simulink model "sampleModel273"  (R2021b)
settings: Solver=VariableStepAuto  StartTime=0.0  StopTime=10.0  RelTol=1e-3
undefined symbols (not defined in the file or in its folder): DiscIntNeverNeededParam
libraries: simulink x13
settings Model: Creator=user  LastModifiedBy=user

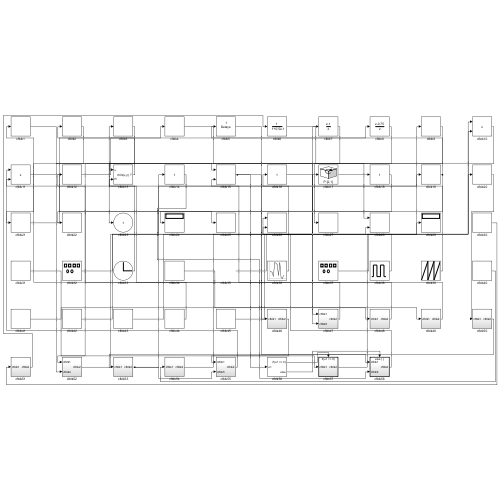
[thumbnail: Simulink's stored preview of the top-level diagram]
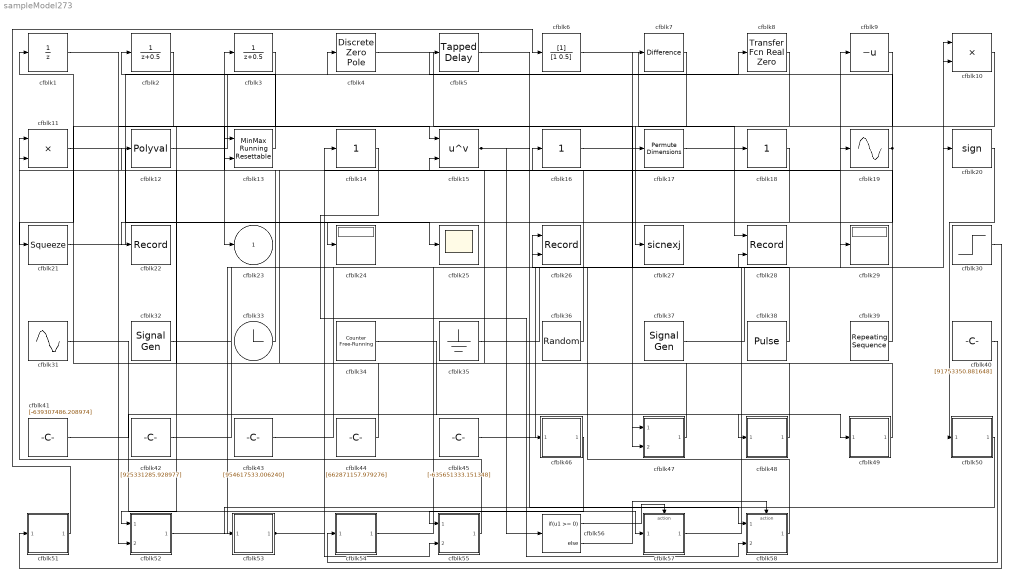
== system sampleModel273 ==
  cfblk1 : UnitDelay  HasFrameUpgradeWarning=on
  cfblk10 : Product
  cfblk11 : Product
  cfblk12 : Polyval  Coefs=[ +2.081618890e-019, -1.441693666e-014, +4.719686976e-010, -8.536869453e-006, +1.621573104e-001, -8.087801117e+001 ]
  cfblk13 : simulink/Math Operations/MinMax Running Resettable  Function=min  vinit=0.0
  cfblk14 : simulink/Math Operations/Slider Gain  gain=1  low=0  high=2
  cfblk15 : Math  Operator=pow  SaturateOnIntegerOverflow=on
  cfblk16 : simulink/Math Operations/Slider Gain  gain=1  low=0  high=2
  cfblk17 : PermuteDimensions
  cfblk18 : simulink/Math Operations/Slider Gain  gain=1  low=0  high=2
  cfblk19 : Sin  TimeSource=Use external signal  SampleTime=0
  cfblk2 : DiscreteTransferFcn  SampleTime=1
  cfblk20 : Signum
  cfblk21 : Squeeze
  cfblk22 : Record  FileSettingsInternal="{\"entries\":[{\"content\":{\"excelSettings\":{\"content\":{},\"type\":\"Streamout.ExcelSettings\"}},\"type\":\"Streamout.FileSettingStorage\",\"uuid\":\"1786dd08-d3d1-48fd-88f3-6c9c5e3b2244\"}],\"packageUris\":[\"http://schema.mathworks.com/mf0/streamout_blocks/R2020a\"],\"version\":\"1.0\"}"  SignalsInternal="{\"entries\":[{\"content\":{\"signals\":[{\"content\":{\"blockPath\":[\"sampleModel273/cfblk22\"],\"channel\":[],\"dimensions\":[1,1],\"domain\":\"sampleModel273/cfblk22\",\"lineColor\":\"#ff13a6\",\"plots\":[1],\"port\":1,\"sid\":[\"\"],\"signalID\":11389,\"signalName\":\"cfblk18\"},\"type\":\"RecordBlkView.Signal\",\"uuid\":\"44d7af05-e021-4219-85f4-b2264b388561\"}]},\"type\":\"RecordBlkView.InputSignals\",\"uuid\":\"1305e598-0f40-4dae-bf49-06488a9adac4\"}],\"packageUris\":[\"http://schema.mathworks.com/mf0/streamout_blocks/R2020a\"],\"version\":\"1.0\"}"  VisualizationBindings="{\"sparklinesplugin\":{\"info\":[{\"bindingParametersList\":[],\"subplotID\":1}]}}"
  cfblk24 : Display
  cfblk25 : Scope
  cfblk26 : Record  FileSettingsInternal="{\"entries\":[{\"content\":{\"excelSettings\":{\"content\":{},\"type\":\"Streamout.ExcelSettings\"}},\"type\":\"Streamout.FileSettingStorage\",\"uuid\":\"c9907c03-a1b4-46c3-905a-7ea5945ed0d3\"}],\"packageUris\":[\"http://schema.mathworks.com/mf0/streamout_blocks/R2020a\"],\"version\":\"1.0\"}"  Layout=[1 1]  SignalsInternal="{\"entries\":[{\"content\":{\"signals\":[{\"content\":{\"blockPath\":[\"sampleModel273/cfblk26\"],\"channel\":[],\"dimensions\":[1],\"domain\":\"sampleModel273/cfblk26\",\"lineColor\":\"#a2142f\",\"plots\":[1],\"port\":1,\"sid\":[\"\"],\"signalID\":11373,\"signalName\":\"cfblk38\"},\"type\":\"RecordBlkView.Signal\",\"uuid\":\"10f35443-25b8-4ed5-9519-77cd749e2a49\"},{\"content\":{\"blockPath\":[\"sampleModel273/cfblk26\"],\"channel\":[],\"dimensions\":[1],\"domain\":\"sampleModel273/cfblk26\",\"lineColor\":\"#139fff\",\"plots\":[1],\"port\":2,\"sid\":[\"\"],\"signalID\":11377,\"signalName\":\"cfblk58\"},\"type\":\"RecordBlkView.Signal\",\"uuid\":\"581304bf-ecf3-443c-9df5-bbc4588b99e1\"}]},\"type\":\"RecordBlkView.InputSignals\",\"uuid\":\"7f34d2d8-bb93-478d-8761-c598979a6e05\"}],\"packageUris\":[\"http://schema.mathworks.com/mf0/streamout_blocks/R2020a\"],\"version\":\"1.0\"}"  VisualizationBindings="{\"xyplotplugin\":{\"info\":[{\"series\":[{\"bindingParametersList\":[{\"parameter\":\"X-Axis\",\"signalID\":11373,\"signalName\":\"cfblk38\"},{\"parameter\":\"Y-Axis\",\"signalID\":11377,\"signalName\":\"cfblk58\"}],\"seriesID\":34757}],\"subplotID\":1}]}}"  CompatibilityTag=XY
  cfblk27 : ToWorkspace  VariableName=sicnexj  SaveFormat=Timeseries  SampleTime=-1
  cfblk28 : Record  FileSettingsInternal="{\"entries\":[{\"content\":{\"excelSettings\":{\"content\":{},\"type\":\"Streamout.ExcelSettings\"}},\"type\":\"Streamout.FileSettingStorage\",\"uuid\":\"f11b4837-361d-47ed-bc23-be4c68ae3fbc\"}],\"packageUris\":[\"http://schema.mathworks.com/mf0/streamout_blocks/R2020a\"],\"version\":\"1.0\"}"  Layout=[1 1]  SignalsInternal="{\"entries\":[{\"content\":{\"signals\":[{\"content\":{\"blockPath\":[\"sampleModel273/cfblk28\"],\"channel\":[],\"dimensions\":[1],\"domain\":\"sampleModel273/cfblk28\",\"lineColor\":\"#a2142f\",\"plots\":[1],\"port\":1,\"sid\":[\"\"],\"signalID\":11381,\"signalName\":\"cfblk6\"},\"type\":\"RecordBlkView.Signal\",\"uuid\":\"39c39639-ba01-4672-b896-9cb9c6ecd09e\"},{\"content\":{\"blockPath\":[\"sampleModel273/cfblk28\"],\"channel\":[],\"dimensions\":[1],\"domain\":\"sampleModel273/cfblk28\",\"lineColor\":\"#139fff\",\"plots\":[1],\"port\":2,\"sid\":[\"\"],\"signalID\":11385,\"signalName\":\"cfblk43\"},\"type\":\"RecordBlkView.Signal\",\"uuid\":\"3ede6f01-830a-4ce5-9876-616c533c0d69\"}]},\"type\":\"RecordBlkView.InputSignals\",\"uuid\":\"89d49a1c-fe7b-4ffb-9ac6-606c9b0ce345\"}],\"packageUris\":[\"http://schema.mathworks.com/mf0/streamout_blocks/R2020a\"],\"version\":\"1.0\"}"  VisualizationBindings="{\"xyplotplugin\":{\"info\":[{\"series\":[{\"bindingParametersList\":[{\"parameter\":\"X-Axis\",\"signalID\":11381,\"signalName\":\"cfblk6\"},{\"parameter\":\"Y-Axis\",\"signalID\":11385,\"signalName\":\"cfblk43\"}],\"seriesID\":55614}],\"subplotID\":1}]}}"  CompatibilityTag=XY
  cfblk29 : Display
  cfblk3 : DiscreteTransferFcn  SampleTime=1
  cfblk30 : Step  Time=[48.000000]  Before=[117438544.028774]  After=[817897715.184338]  SampleTime=0
  cfblk31 : Sin  Amplitude=[629555870.349999]  Bias=[755274726.941135]  SampleTime=0
  cfblk32 : SignalGenerator  WaveForm=square  Amplitude=[-783473337.137861]
  cfblk33 : Clock
  cfblk34 : simulink/Sources/Counter Free-Running  NumBits=[52.000000]  tsamp=-1
  cfblk35 : Ground
  cfblk36 : RandomNumber  Mean=[98921.584735]  Variance=[34184.174299]  Seed=[249651186.000000]  SampleTime=0.1
  cfblk37 : SignalGenerator  Amplitude=[196507773.243477]
  cfblk38 : DiscretePulseGenerator  PulseType=Time based  Amplitude=[376878024.596685]  Period=[65768725.640575]  PulseWidth=5  PhaseDelay=[3.000000]
  cfblk39 : simulink/Sources/Repeating Sequence  rep_seq_t=[0 2]  rep_seq_y=[-584950579.786823, 340676402.746707]
  cfblk4 : DiscreteZeroPole  Poles=[0 0.5]  Gain=1
  cfblk40 : Constant  Value=[91753350.881648]  SampleTime=1
  cfblk41 : Constant  Value=[-639307486.208974]  SampleTime=1
  cfblk42 : Constant  Value=[925331285.928977]  SampleTime=1
  cfblk43 : Constant  Value=[954617533.006240]  SampleTime=1
  cfblk44 : Constant  Value=[662871157.979276]  SampleTime=1
  cfblk45 : Constant  Value=[-635651333.151348]  SampleTime=1
  cfblk46 : Subsystem
  cfblk47 : Subsystem
  cfblk48 : Subsystem
  cfblk49 : Subsystem
  cfblk5 : simulink/Discrete/Tapped Delay  vinit=0.0  samptime=-1  NumDelays=1  DelayOrder=Oldest  includeCurrent=off
  cfblk50 : Subsystem
  cfblk51 : Subsystem
  cfblk52 : Subsystem
  cfblk53 : Subsystem
  cfblk54 : Subsystem
  cfblk55 : Subsystem
  cfblk56 : If  IfExpression=u1 >= 0  SampleTime=1
  cfblk57 : Subsystem  TreatAsAtomicUnit=on
  cfblk58 : Subsystem  TreatAsAtomicUnit=on
  cfblk6 : DiscreteFilter  SampleTime=1
  cfblk7 : simulink/Discrete/Difference  ICPrevInput=0.0  OutMin=[]  OutMax=[]  OutDataTypeStr=Inherit: Inherit via back propagation  OutDataType=fixdt(1, 16)  OutScaling=2^-10  DoSatur=off
  cfblk8 : simulink/Discrete/Transfer Fcn Real Zero  ZeroZ=0.75  ICPrevInput=0.0  DoSatur=off
      settings: SourceProductBaseCode=SL
  cfblk9 : UnaryMinus
  cfblk23 : Outport
  wires:
  cfblk8/1 -> cfblk23/1
  cfblk36/1 -> cfblk16/1
  cfblk19/1 -> cfblk24/1, cfblk5/1
  cfblk55/1(cfblk2) -> cfblk11/1
  cfblk57/1(cfblk2) -> cfblk10/1
  cfblk9/1 -> cfblk21/1
  cfblk17/1 -> cfblk18/1
  cfblk44/1 -> cfblk1/1
  cfblk21/1 -> cfblk4/1
  cfblk15/1 -> cfblk58/1(cfblk1), cfblk56/1
  cfblk12/1 -> cfblk8/1
  cfblk14/1 -> cfblk58/2(cfblk5)
  cfblk33/1 -> cfblk3/1
  cfblk37/1 -> cfblk9/1
  cfblk11/1 -> cfblk25/1
  cfblk10/1 -> cfblk27/1
  cfblk20/1 -> cfblk50/1(cfblk1)
  cfblk13/1 -> cfblk2/1
  cfblk52/1(cfblk2) -> cfblk14/1
  cfblk18/1 -> cfblk22/1
  cfblk3/1 -> cfblk52/1(cfblk1)
  cfblk1/1 -> cfblk15/1
  cfblk54/1(cfblk2) -> cfblk10/2
  cfblk35/1 -> cfblk17/1
  cfblk38/1 -> cfblk26/1
  cfblk2/1 -> cfblk52/2(cfblk4)
  cfblk7/1 -> cfblk13/1
  cfblk40/1 -> cfblk54/1(cfblk1)
  cfblk50/1(cfblk2) -> cfblk53/1(cfblk1)
  cfblk6/1 -> cfblk28/1
  cfblk48/1(cfblk2) -> cfblk15/2
  cfblk53/1(cfblk2) -> cfblk19/1, cfblk55/2(cfblk5)
  cfblk45/1 -> cfblk29/1
  cfblk5/1 -> cfblk46/1(cfblk1)
  cfblk42/1 -> cfblk7/1
  cfblk31/1 -> cfblk57/1(cfblk1)
  cfblk41/1 -> cfblk48/1(cfblk1)
  cfblk34/1 -> cfblk49/1(cfblk1)
  cfblk47/1(cfblk2) -> cfblk12/1
  cfblk43/1 -> cfblk28/2
  cfblk58/1(cfblk2) -> cfblk26/2
  cfblk30/1 -> cfblk51/1(cfblk1)
  cfblk32/1 -> cfblk20/1
  cfblk39/1 -> cfblk11/2
  cfblk49/1(cfblk2) -> cfblk13/2
  cfblk16/1 -> cfblk47/1(cfblk1)
  cfblk46/1(cfblk2) -> cfblk55/1(cfblk1)
  cfblk4/1 -> cfblk47/2(cfblk5)
  cfblk51/1(cfblk2) -> cfblk6/1
  cfblk56/1 -> cfblk57/Action
  cfblk56/2 -> cfblk58/Action

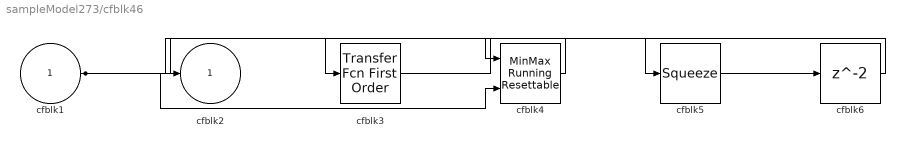
== system sampleModel273/cfblk46 ==
  cfblk1 : Inport
  cfblk3 : simulink/Discrete/Transfer Fcn First Order  PoleZ=0.95  ICPrevOutput=0.0  DoSatur=off
  cfblk4 : simulink/Math Operations/MinMax Running Resettable  Function=min  vinit=0.0
  cfblk5 : Squeeze
  cfblk6 : Delay  SampleTime=1
  cfblk2 : Outport
  wires:
  cfblk3/1 -> cfblk5/1
  cfblk1/1 -> cfblk4/1, cfblk4/2
  cfblk4/1 -> cfblk2/1
  cfblk5/1 -> cfblk6/1
  cfblk6/1 -> cfblk3/1

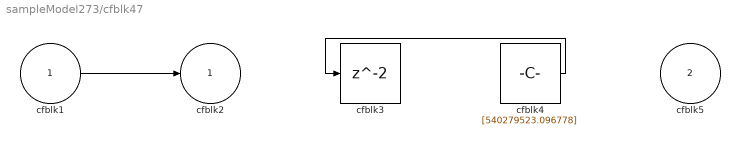
== system sampleModel273/cfblk47 ==
  cfblk1 : Inport
  cfblk5 : Inport  Port=2
  cfblk3 : Delay  SampleTime=1
  cfblk4 : Constant  Value=[540279523.096778]  SampleTime=1
  cfblk2 : Outport
  wires:
  cfblk4/1 -> cfblk3/1
  cfblk1/1 -> cfblk2/1

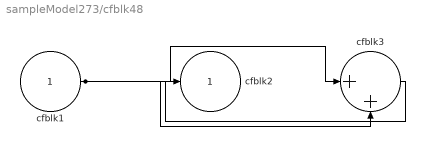
== system sampleModel273/cfblk48 ==
  cfblk1 : Inport
  cfblk3 : Sum  Inputs=|++
  cfblk2 : Outport
  wires:
  cfblk1/1 -> cfblk3/1, cfblk3/2
  cfblk3/1 -> cfblk2/1

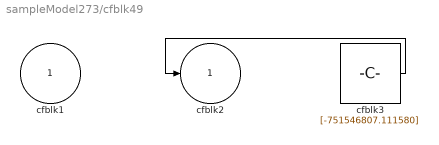
== system sampleModel273/cfblk49 ==
  cfblk1 : Inport
  cfblk3 : Constant  Value=[-751546807.111580]  SampleTime=1
  cfblk2 : Outport
  wires:
  cfblk3/1 -> cfblk2/1

== system sampleModel273/cfblk50 ==
  cfblk1 : Inport
  cfblk3 : Constant  Value=[-904146533.282916]  SampleTime=1
  cfblk2 : Outport
  wires:
  cfblk1/1 -> cfblk2/1

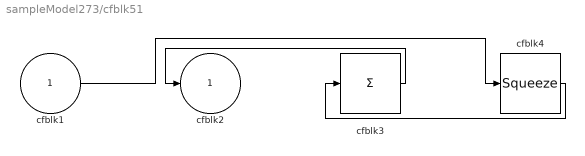
== system sampleModel273/cfblk51 ==
  cfblk1 : Inport
  cfblk3 : Sum  Inputs=+
  cfblk4 : Squeeze
  cfblk2 : Outport
  wires:
  cfblk3/1 -> cfblk2/1
  cfblk4/1 -> cfblk3/1
  cfblk1/1 -> cfblk4/1

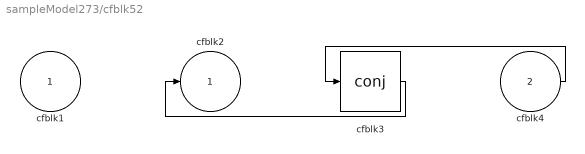
== system sampleModel273/cfblk52 ==
  cfblk1 : Inport
  cfblk4 : Inport  Port=2
  cfblk3 : Math  Operator=conj  SaturateOnIntegerOverflow=on
  cfblk2 : Outport
  wires:
  cfblk4/1 -> cfblk3/1
  cfblk3/1 -> cfblk2/1

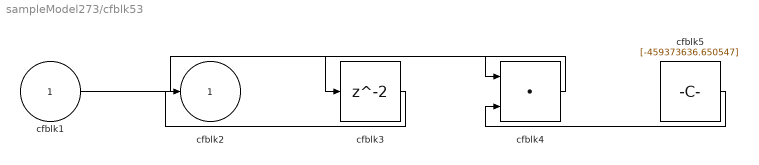
== system sampleModel273/cfblk53 ==
  cfblk1 : Inport
  cfblk3 : Delay  SampleTime=1
  cfblk4 : DotProduct  InputSameDT=on  OutDataTypeStr=Inherit: Inherit via internal rule
  cfblk5 : Constant  Value=[-459373636.650547]  SampleTime=1
  cfblk2 : Outport
  wires:
  cfblk1/1 -> cfblk4/1
  cfblk3/1 -> cfblk2/1
  cfblk5/1 -> cfblk4/2
  cfblk4/1 -> cfblk3/1

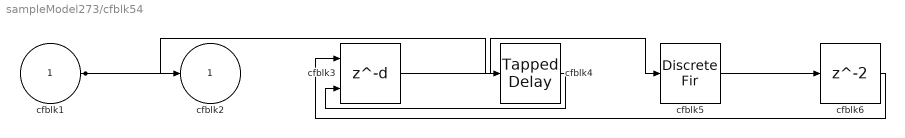
== system sampleModel273/cfblk54 ==
  cfblk1 : Inport
  cfblk3 : Delay  DelayLengthSource=Input port  SampleTime=1
      settings: InputPortMap=u0,p1
  cfblk4 : simulink/Discrete/Tapped Delay  vinit=0.0  samptime=-1  NumDelays=1  DelayOrder=Oldest  includeCurrent=off
  cfblk5 : DiscreteFir  SampleTime=1
  cfblk6 : Delay  SampleTime=1
  cfblk2 : Outport
  wires:
  cfblk1/1 -> cfblk2/1, cfblk4/1
  cfblk4/1 -> cfblk3/2
  cfblk3/1 -> cfblk5/1
  cfblk5/1 -> cfblk6/1
  cfblk6/1 -> cfblk3/1

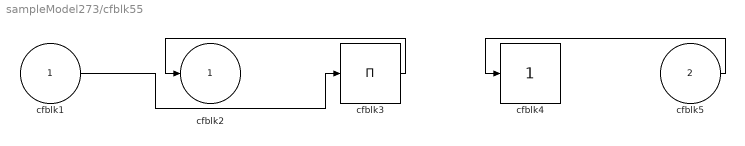
== system sampleModel273/cfblk55 ==
  cfblk1 : Inport
  cfblk5 : Inport  Port=2
  cfblk3 : Product  Inputs=*
  cfblk4 : simulink/Math Operations/Slider Gain  gain=1  low=0  high=2
  cfblk2 : Outport
  wires:
  cfblk5/1 -> cfblk4/1
  cfblk3/1 -> cfblk2/1
  cfblk1/1 -> cfblk3/1

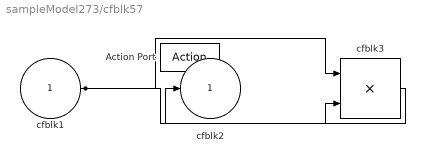
== system sampleModel273/cfblk57 ==
  cfblk1 : Inport
  Action Port : ActionPort  ActionPortLabel=if(u1 >= 0)
  cfblk3 : Product  Inputs=**
  cfblk2 : Outport
  wires:
  cfblk3/1 -> cfblk2/1
  cfblk1/1 -> cfblk3/1, cfblk3/2

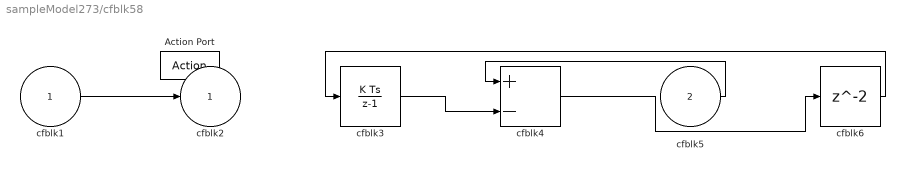
== system sampleModel273/cfblk58 ==
  cfblk1 : Inport
  cfblk5 : Inport  Port=2
  Action Port : ActionPort  ActionPortLabel=else
  cfblk3 : DiscreteIntegrator  SampleTime=-1  ICPrevOutput=DiscIntNeverNeededParam  ICPrevScaledInput=DiscIntNeverNeededParam
  cfblk4 : Sum  Inputs=+-
  cfblk6 : Delay
  cfblk2 : Outport
  wires:
  cfblk5/1 -> cfblk4/1
  cfblk3/1 -> cfblk4/2
  cfblk1/1 -> cfblk2/1
  cfblk4/1 -> cfblk6/1
  cfblk6/1 -> cfblk3/1
